simulink model "test_single_phase_diode_rectifier"  (R2017b)
settings: Solver=ode4  StartTime=0.0  StopTime=0.02  FixedStep=1e-6  MaxStep=1e-4  RelTol=1e-3
libraries: powerlib x5, typhoonHILlib x1
settings Model: Creator=Marcos  LastModifiedBy=Marcos

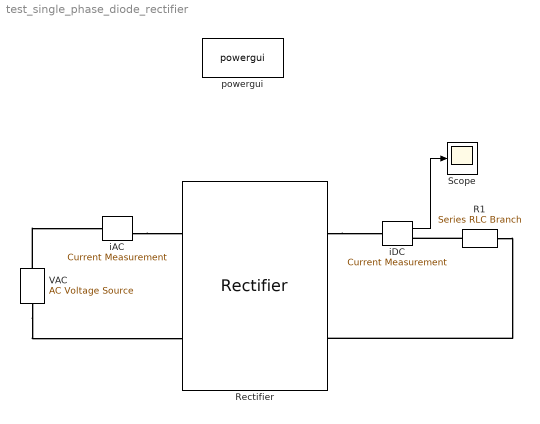
== system test_single_phase_diode_rectifier ==
  R1 : powerlib/Elements/Series RLC Branch  LConnTagsString=__new0  RConnTagsString=__new0  BranchType=R  Resistance=10  Inductance=1e-3  SetiL0=off  InitialCurrent=0  Capacitance=1e-6  Setx0=off  InitialVoltage=0  Measurements=None
  Rectifier : typhoonHILlib/Rectifier  RecType=Diode  ThreePhase=off  sa_top_logic=Active-high  sa_bot_logic=Active-high  sb_top_logic=Active-high  sb_bot_logic=Active-high  sc_top_logic=Active-high  sc_bot_logic=Active-high  di_sa_top=1  di_sa_bot=2  di_sb_top=3  di_sb_bot=4  di_sc_top=5  di_sc_bot=6  v_sa_top=off  i_sa_top=off  v_sa_bot=off  i_sa_bot=off  v_sb_top=off  i_sb_top=off  v_sb_bot=off  i_sb_bot=off  v_sc_top=off  i_sc_top=off  v_sc_bot=off  i_sc_bot=off  r_on=0.001  v_f=0  r_s=1e4  c_s=inf  toggle_init=on  toggle_draw=on  model_loaded=off  old_pat=typhoonPatterns/Diode Rectifier (1-Phase)  old_size=145,209
      settings: SourceProductName=Typhoon HIL
  Scope : Scope
  VAC : powerlib/Electrical Sources/AC Voltage Source  Amplitude=311.123  Phase=0  Frequency=50  SampleTime=0  Measurements=None  BusType=swing  Pref=10e3  Qref=0  Qmin=-inf  Qmax=+inf
  iAC : powerlib/Measurements/Current Measurement  PhasorSimulation=off  OutputType=Complex  PSBequivalent=0
  iDC : powerlib/Measurements/Current Measurement  PhasorSimulation=off  OutputType=Complex  PSBequivalent=0
  powergui : powerlib/powergui  Priority=1  SimulationMode=Continuous  SampleTime=10e-6  frequency=60  Iterations=50  frequencyindice=50  Pbase=100e6  ErrMax=1e-4  UnitsV=kV  UnitsW=MW  buscounter=0  FunctionMessages=off  echomessages=off  EnableUseOfTLC=off  CurrentSourceSwitches=off  DisableSnubberDevices=off  DisableRonSwitches=off  DisableVfSwitches=off  DisplayEquations=off  SolverType=Tustin/Backward Euler (TBE)  Interpol=off  ExternalGateDelay=off  methode=off  Ts=100  x0status=blocks  SPID=on  SwTol=0  HookPort=off  RestoreLinks=warning  ResistiveCurrentMeasurement=off  Frange=[0:2:500]  Ylog=off  Xlog=on  ShowGrid=off  save=off  variable=ZData  structure=0  ZoomFFT=off  StartTime=0.0  cycles=1  DisplayStyle=1  fundamental=60  FreqAxis=off  MaxFrequency=1000  frequencyindicesteady=1  RmsSteady=1  display=off
  wires:
  iDC/1 -> Scope/1
  connections:
  R1/LConn1 -- iDC/RConn1
  Rectifier/RConn1 -- iDC/LConn1
  R1/RConn1 -- Rectifier/RConn2
  iAC/RConn1 -- Rectifier/LConn1
  VAC/RConn1 -- iAC/LConn1
  VAC/LConn1 -- Rectifier/LConn2
